simulink library "lib_Convection_ImpingingJet"  (R2015a)
settings: Solver=ode45  StartTime=0.0  StopTime=10.0  RelTol=1e-3
libraries: simulink x35, lib_GenTools_MinMax x1
settings Model: Creator=jlkratz  LastModifiedBy=jlkratz

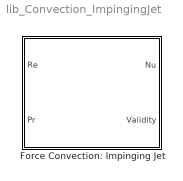
== system lib_Convection_ImpingingJet ==
  Force Convection: Impinging Jet : Subsystem  mask(TSAT: Impinging Jet){RoundOrSlot_M=Slot Nozzle, SingleOrArray_M=Nozzle Array, AlignOrStag_M=Nozzles are aligned, H_M=0.126/12, D_M=0.0625/12, r_M=3, S_M=0.25/12}
      mask prompts: H_M "H_M - Distance from the nozzle to the impingement surface (H)"; D_M "D_M - Diameter of the nozzle (D) for round nozzles or the width of the slot nozzle (W) for slot nozzles"; r_M "r_M - Distance from the stagnation point over which the average Nu is desired (r or x)"; S_M "S_M - Pitch of the array (distance between centerpoints the nozzles in an array)"
      mask help:
      | This block estimates the average Nusselt number for an impinging jet on a surfaces. The implemented correlations were developed by Martin. It is presumed in these correlations that the gas jet exits its nozzle with a uniform velocity, temperature, and species concentration. Thermal and compositional equilibrium with the ambient air are presumed. Conditions are assumed to be uninfluenced by the amount of turbulence at the nozzles and the surface is presumed to be stationary. Fluid properties should be evaluated at the conditions of the jet. This block considers round nozzles, and slot nozzles. It also considers a single nozzle or an array of nozzles. The characteristic length is the hydraulic diameter of the nozzle which happens to be the diameter (D) for round nozzles and 2 times the width of the slot (W) for slot nozzles. The implemented correlations are subject to the following restrictions:
      |
      | Single Round Nozzle:
      | 2000 <= Re <= 400000
      | 2 <= H/D <= 12
      | 0.004 <= Ar <= 0.04
      |
      | Array of Round Nozzles:
      | 2000 <= Re <= 100000
      | 2 <= H/D <= 12
      | 0.004 <= Ar <= 0.04
      |
      | Single Slot Nozzle:
      | 3000 <= Re <= 90000
      | 2 <= H/W <= 10
      | 0.025 <= Ar <= 0.125
      |
      | Array of Slot Nozzles:
      | 1500 <= Re <= 40000
      | 2 <= H/W <= 80
      | 0.008 <= Ar <= 2.5*Aro (Aro is defined in the help menu)
      |
      | Note that Re is the Reynolds number, Pr is the Prandtl number, H is the distance from the nozzle to the impingment surface, and Ar is a nozzle ratio (the nozzle exit area to the surface area of the cell). For a single nozzle the cell is defined by a radius or distance from the stagnation point which defines the area over which the average Nusselt number is to be calculated for. For nozzle areas, the cell area is equally divided area in which each nozzle resides. For more information see the block help menu.
      mask Help: web(which('Convection_TSAT_ImpingingJet.html'),'-helpbrowser')
      mask TypeOptions RoundOrSlot_M: Round Nozzle | Slot Nozzle
      mask Callback RoundOrSlot_M:
      | sel1 = get_param(gcb,'RoundOrSlot_M');
      | sel2 = get_param(gcb,'SingleOrArray_M');
      | if sel2(1) == 'N'
      |     if sel1(1) == 'R'
      |         MSK_SEC_Enables3_TSAT('on',[3],'en')
      |     elseif sel1(1) == 'S'
      |         MSK_SEC_Enables3_TSAT('on',[3],'dis')
      |     end
      | end
      | clear sel1 sel2
      mask TypeOptions SingleOrArray_M: Single Nozzle | Nozzle Array
      mask Callback SingleOrArray_M:
      | sel1 = get_param(gcb,'SingleOrArray_M');
      | sel2 = get_param(gcb,'RoundOrSlot_M');
      | if sel1(1) == 'S'
      |     MSK_SEC_Enables3_TSAT('on',7,'dis')
      |     MSK_SEC_Enables3_TSAT('on',6,'en')
      |     MSK_SEC_Enables3_TSAT('on',3,'dis')
      | elseif sel1(1) == 'N'
      |     MSK_SEC_Enables3_TSAT('on',7,'en')
      |     MSK_SEC_Enables3_TSAT('on',6,'dis')
      |     if sel2(1) == 'R'
      |         MSK_SEC_Enables3_TSAT('on',3,'en')
      |     elseif sel2(1) == 'S'
      |         MSK_SEC_Enables3_TSAT('on',3,'dis')
      |     end
      | end
      | clear sel1 sel2
      mask TypeOptions AlignOrStag_M: Nozzles are aligned | Nozzles are staggered
      mask DialogControl Container3 Prompt: Parameters

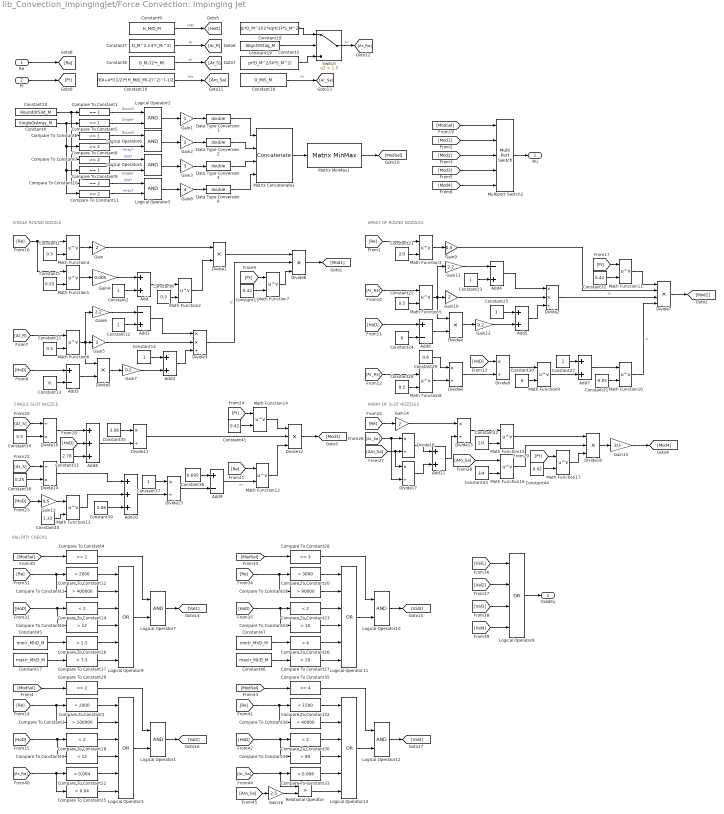
== system lib_Convection_ImpingingJet/Force Convection: Impinging Jet ==
  note: SINGLE ROUND NOZZLE
  note: SINGLE SLOT NOZZLE
  note: ARRAY OF ROUND NOZZLES
  note: ARRAY OF SLOT NOZZLES
  note: VALIDITY CHECKS
  Re : Inport
  Pr : Inport  Port=2
  Add{,2,5,7,11} (5 alike) : Sum
  Add1 : Sum  Inputs=-+
  Add10 : Sum  Inputs=+++
  Add3 : Sum  Inputs=+-
  Add4 : Sum  Inputs=-+
  Add6 : Sum  Inputs=+-
  Add8 : Sum  Inputs=+++
  Add9 : Sum  Inputs=+-
  Compare To Constant{1,4..6,9} (5 alike) : simulink/Logic and Bit Operations/Compare To Constant  relop===  const=1  OutDataTypeStr=boolean
  Compare To Constant{7..8,10..11,29} (5 alike) : simulink/Logic and Bit Operations/Compare To Constant  relop===  const=2  OutDataTypeStr=boolean
  Compare To Constant12 : simulink/Logic and Bit Operations/Compare To Constant  relop=<  const=2000  OutDataTypeStr=boolean
  Compare To Constant13 : simulink/Logic and Bit Operations/Compare To Constant  relop=>  const=400000  OutDataTypeStr=boolean
  Compare To Constant{14,18,23,30} (4 alike) : simulink/Logic and Bit Operations/Compare To Constant  relop=<  const=2  OutDataTypeStr=boolean
  Compare To Constant15 : simulink/Logic and Bit Operations/Compare To Constant  relop=>  const=12  OutDataTypeStr=boolean
  Compare To Constant16 : simulink/Logic and Bit Operations/Compare To Constant  relop=<  const=2.5  OutDataTypeStr=boolean
  Compare To Constant17 : simulink/Logic and Bit Operations/Compare To Constant  relop=>  const=7.5  OutDataTypeStr=boolean
  Compare To Constant19 : simulink/Logic and Bit Operations/Compare To Constant  relop=>  const=12  OutDataTypeStr=boolean
  Compare To Constant2 : simulink/Logic and Bit Operations/Compare To Constant  relop=<  const=2000  OutDataTypeStr=boolean
  Compare To Constant20 : simulink/Logic and Bit Operations/Compare To Constant  relop=<  const=3000  OutDataTypeStr=boolean
  Compare To Constant21 : simulink/Logic and Bit Operations/Compare To Constant  relop=>  const=90000  OutDataTypeStr=boolean
  Compare To Constant22 : simulink/Logic and Bit Operations/Compare To Constant  relop=<  const=0.004  OutDataTypeStr=boolean
  Compare To Constant24 : simulink/Logic and Bit Operations/Compare To Constant  relop=>  const=10  OutDataTypeStr=boolean
  Compare To Constant25 : simulink/Logic and Bit Operations/Compare To Constant  relop=>  const=0.04  OutDataTypeStr=boolean
  Compare To Constant26 : simulink/Logic and Bit Operations/Compare To Constant  relop=<  const=4  OutDataTypeStr=boolean
  Compare To Constant27 : simulink/Logic and Bit Operations/Compare To Constant  relop=>  const=20  OutDataTypeStr=boolean
  Compare To Constant28 : simulink/Logic and Bit Operations/Compare To Constant  relop===  const=3  OutDataTypeStr=boolean
  Compare To Constant3 : simulink/Logic and Bit Operations/Compare To Constant  relop=>  const=100000  OutDataTypeStr=boolean
  Compare To Constant31 : simulink/Logic and Bit Operations/Compare To Constant  relop=>  const=80  OutDataTypeStr=boolean
  Compare To Constant32 : simulink/Logic and Bit Operations/Compare To Constant  relop=<  const=1500  OutDataTypeStr=boolean
  Compare To Constant33 : simulink/Logic and Bit Operations/Compare To Constant  relop=<  const=0.008  OutDataTypeStr=boolean
  Compare To Constant35 : simulink/Logic and Bit Operations/Compare To Constant  relop===  const=4  OutDataTypeStr=boolean
  Compare To Constant36 : simulink/Logic and Bit Operations/Compare To Constant  relop=>  const=40000  OutDataTypeStr=boolean
  Constant{1,6,11,22,28,34} (6 alike) : Constant  Value=0.5
  Constant10 : Constant  Value=(60+4*((1/2)*(H_M/D_M)-2)^2)^(-1/2)
  Constant{2,12,14,23,25,27,37} (7 alike) : Constant
  Constant13 : Constant  Value=6
  Constant{15,32,41,44} (4 alike) : Constant  Value=0.42
  Constant16 : Constant  Value=D_M/S_M
  Constant17 : Constant  Value=max(r_M)/D_M
  Constant18 : Constant  Value=pi*D_M^2/(2*sqrt(3)*S_M^2)
  Constant19 : Constant  Value=AlignOrStag_M
  Constant20 : Constant  Value=RoundOrSlot_M
  Constant21 : Constant  Value=2/3
  Constant24 : Constant  Value=6
  Constant29 : Constant  Value=0.6
  Constant3 : Constant  Value=pi*D_M^2/(4*S_M^2)
  Constant30 : Constant  Value=6
  Constant31 : Constant  Value=-0.05
  Constant33 : Constant  Value=2.78
  Constant35 : Constant  Value=3.06
  Constant36 : Constant  Value=0.695
  Constant38 : Constant  Value=0.25
  Constant39 : Constant  Value=3.06
  Constant4 : Constant  Value=SingleOrArray_M
  Constant40 : Constant  Value=1.33
  Constant42 : Constant  Value=2/3
  Constant43 : Constant  Value=3/4
  Constant45 : Constant  Value=min(r_M)/D_M
  Constant46 : Constant  Value=max(r_M)/D_M
  Constant47 : Constant  Value=min(r_M)/D_M
  Constant5 : Constant  Value=0.55
  Constant7 : Constant  Value=D_M^2./(4*r_M.^2)
  Constant8 : Constant  Value=D_M./(2*r_M)
  Constant9 : Constant  Value=H_M/D_M
  Data Type Conversion{1..3,8} (4 alike) : DataTypeConversion  OutDataTypeStr=double
  Divide1 : Product  Inputs=**
  Divide10 : Product  Inputs=/*
  Divide{8..9,11,13,15..17} (7 alike) : Product  Inputs=*/
  Divide12 : Product  Inputs=***
  Divide14 : Product  Inputs=/*
  Divide18 : Product  Inputs=***
  Divide2 : Product  Inputs=**/
  Divide3 : Product  Inputs=**/
  Divide4 : Product  Inputs=**
  Divide5 : Product  Inputs=**
  Divide6 : Product  Inputs=***
  Divide7 : Product  Inputs=****
  Gain{,2,5,10,14} (5 alike) : Gain  Gain=2
  Gain1 : Gain
  Gain11 : Gain  Gain=2.2
  Gain12 : Gain  Gain=0.2
  Gain13 : Gain  Gain=0.5
  Gain15 : Gain  Gain=2/3
  Gain16 : Gain  Gain=2.5
  Gain3 : Gain  Gain=3
  Gain4 : Gain  Gain=0.005
  Gain6 : Gain  Gain=2.2
  Gain7 : Gain  Gain=0.2
  Gain8 : Gain  Gain=4
  Gain9 : Gain  Gain=0.5
  Logical Operator{1..2,4..7,10,12} (8 alike) : Logic  AllPortsSameDT=off  OutDataTypeStr=boolean
  Logical Operator{3,9,11,13} (4 alike) : Logic  Operator=OR  Inputs=6  AllPortsSameDT=off  OutDataTypeStr=boolean
  Logical Operator8 : Logic  Operator=OR  Inputs=4  AllPortsSameDT=off  OutDataTypeStr=boolean
  Math Function{1..17} (17 alike) : Math  Operator=pow  SaturateOnIntegerOverflow=on
  Matrix Concatenate1 : Concatenate  NumInputs=4  Mode=Multidimensional array  ConcatenateDimension=2
  Matrix MinMax1 : lib_GenTools_MinMax/Matrix MinMax  rows_M=on  cols_M=off  all_M=off  minmax_M=off  BN_M=gcb
  Multiport Switch2 : MultiPortSwitch  Inputs=4
  Relational Operator : RelationalOperator  Operator=>  OutDataTypeStr=boolean
  Switch : Switch  Criteria=u2 > Threshold  Threshold=1.5
  Nu : Outport
  Validity : Outport  Port=2
  wires:
  Gain16/1 -> Relational Operator/2
  Constant1/1 -> Math Function4/2
  Re/1 -> [Re]
  Pr/1 -> [Pr]
  [ModSel] -> Multiport Switch2/1
  Multiport Switch2/1 -> Nu/1
  Matrix MinMax1/1 -> [ModSel]
  Matrix Concatenate1/1 -> Matrix MinMax1/1
  [Re] -> Math Function1/1, Math Function4/1
  Gain1/1 -> Data Type Conversion1/1
  Logical Operator2/1 -> Gain1/1
  Gain2/1 -> Data Type Conversion2/1
  Logical Operator6/1 -> Gain2/1
  Gain3/1 -> Data Type Conversion3/1
  Logical Operator4/1 -> Gain3/1
  Gain8/1 -> Data Type Conversion8/1
  Logical Operator5/1 -> Gain8/1
  Data Type Conversion1/1 -> Matrix Concatenate1/1
  Data Type Conversion2/1 -> Matrix Concatenate1/2
  Data Type Conversion3/1 -> Matrix Concatenate1/3
  Data Type Conversion8/1 -> Matrix Concatenate1/4
  Constant20/1 -> Compare To Constant10/1, Compare To Constant7/1, Compare To Constant6/1, Compare To Constant1/1
  Constant4/1 -> Compare To Constant11/1, Compare To Constant9/1, Compare To Constant8/1, Compare To Constant5/1
  Compare To Constant1/1 -> Logical Operator2/1  "Round?"
  Compare To Constant5/1 -> Logical Operator2/2  "Single?"
  Compare To Constant6/1 -> Logical Operator6/1  "Round?"
  Compare To Constant8/1 -> Logical Operator6/2  "Array?"
  Compare To Constant7/1 -> Logical Operator4/1  "Slot?"
  Compare To Constant9/1 -> Logical Operator4/2  "Single?"
  Compare To Constant10/1 -> Logical Operator5/1  "Slot?"
  Compare To Constant11/1 -> Logical Operator5/2  "Array?"
  [Mod1] -> Multiport Switch2/2
  [Mod2] -> Multiport Switch2/3
  [Mod3] -> Multiport Switch2/4
  [Mod4] -> Multiport Switch2/5
  Math Function4/1 -> Gain/1
  Constant2/1 -> Add/2
  Constant5/1 -> Math Function1/2
  Math Function1/1 -> Gain4/1
  Gain4/1 -> Add/1
  Add/1 -> Math Function2/1
  Constant6/1 -> Math Function2/2
  Math Function2/1 -> Divide1/2
  Gain/1 -> Divide1/1
  Constant7/1 -> [Ar_R]  "Ar"
  Constant8/1 -> [Ar_S]  "Ar"
  Constant9/1 -> [HoD]  "H/D"
  Constant10/1 -> [Aro_Sa]  "Aro"
  [Ar_R] -> Math Function6/1
  Constant11/1 -> Math Function6/2
  Math Function6/1 -> Divide5/1, Gain6/1, Gain5/1
  Constant12/1 -> Add1/2
  Gain6/1 -> Add1/1
  Gain5/1 -> Divide3/2
  Add1/1 -> Divide3/1
  [HoD] -> Add3/1
  Constant13/1 -> Add3/2
  Add3/1 -> Divide5/2
  Divide5/1 -> Gain7/1
  Gain7/1 -> Add2/2
  Constant14/1 -> Add2/1
  Add2/1 -> Divide3/3
  Divide1/1 -> Divide6/1
  Divide3/1 -> Divide6/2  "G"
  [Pr] -> Math Function7/1
  Math Function7/1 -> Divide6/3
  Constant15/1 -> Math Function7/2
  Divide6/1 -> [Mod1]
  Constant16/1 -> [Ar_Sa]  "Ar"
  Constant3/1 -> Switch/3
  Constant18/1 -> Switch/1
  Switch/1 -> [Ar_Ra]  "Ar"
  Constant19/1 -> Switch/2
  Constant21/1 -> Math Function3/2
  [Re] -> Math Function3/1
  Math Function3/1 -> Gain9/1
  Gain9/1 -> Divide7/2
  [Ar_Ra] -> Math Function5/1
  Constant22/1 -> Math Function5/2
  Math Function5/1 -> Gain10/1, Gain11/1, Divide4/1
  Constant23/1 -> Add4/2
  Gain11/1 -> Add4/1
  Gain10/1 -> Divide2/2
  Add4/1 -> Divide2/1
  [HoD] -> Add6/1
  Add6/1 -> Divide4/2
  Divide4/1 -> Gain12/1
  Gain12/1 -> Add5/2
  Constant25/1 -> Add5/1
  Add5/1 -> Divide2/3
  Divide2/1 -> Divide7/3  "G"
  Constant24/1 -> Add6/2
  Math Function9/1 -> Add7/2
  Constant27/1 -> Add7/1
  [Ar_Ra] -> Math Function8/1
  Constant28/1 -> Math Function8/2
  Math Function8/1 -> Divide8/2
  Constant29/1 -> Divide8/1
  Divide8/1 -> Divide9/2
  [HoD] -> Divide9/1
  Divide9/1 -> Math Function9/1
  Constant30/1 -> Math Function9/2
  Add7/1 -> Math Function10/1
  Constant31/1 -> Math Function10/2
  Math Function10/1 -> Divide7/4  "K"
  Divide7/1 -> [Mod2]
  [Pr] -> Math Function11/1
  Math Function11/1 -> Divide7/1
  Constant32/1 -> Math Function11/2
  Constant34/1 -> Divide10/2
  [Ar_S] -> Divide10/1
  Divide10/1 -> Add8/1
  [HoD] -> Add8/2
  Constant33/1 -> Add8/3
  Add8/1 -> Divide11/2
  Constant35/1 -> Divide11/1
  [Re] -> Math Function12/1
  Add9/1 -> Math Function12/2  "m"
  Divide11/1 -> Divide12/2
  Math Function12/1 -> Divide12/3
  Divide12/1 -> [Mod3]
  Constant37/1 -> Divide13/1
  Constant36/1 -> Add9/1
  Divide13/1 -> Add9/2
  Add10/1 -> Divide13/2
  Constant38/1 -> Divide14/2
  [Ar_S] -> Divide14/1
  Constant39/1 -> Add10/3
  Divide14/1 -> Add10/1
  [HoD] -> Gain13/1
  Gain13/1 -> Math Function13/1
  Constant40/1 -> Math Function13/2
  Math Function13/1 -> Add10/2
  [Pr] -> Math Function14/1
  Math Function14/1 -> Divide12/1
  Constant41/1 -> Math Function14/2
  [Re] -> Gain14/1
  [Ar_Sa] -> Divide17/2, Divide16/1
  [Aro_Sa] -> Divide17/1, Divide16/2
  Divide16/1 -> Add11/1
  Divide17/1 -> Add11/2
  Gain14/1 -> Divide15/1
  Add11/1 -> Divide15/2
  Divide15/1 -> Math Function15/1
  Constant42/1 -> Math Function15/2
  [Aro_Sa] -> Math Function16/1
  Constant43/1 -> Math Function16/2
  Math Function15/1 -> Divide18/1
  Math Function16/1 -> Divide18/2
  [Pr] -> Math Function17/1
  Constant44/1 -> Math Function17/2
  Math Function17/1 -> Divide18/3
  Divide18/1 -> Gain15/1
  Gain15/1 -> [Mod4]
  [Re] -> Compare To Constant13/1, Compare To Constant12/1
  [HoD] -> Compare To Constant15/1, Compare To Constant14/1
  Constant45/1 -> Compare To Constant16/1
  Constant17/1 -> Compare To Constant17/1
  Compare To Constant16/1 -> Logical Operator9/5
  Compare To Constant17/1 -> Logical Operator9/6
  Compare To Constant15/1 -> Logical Operator9/4
  Compare To Constant14/1 -> Logical Operator9/3
  Compare To Constant13/1 -> Logical Operator9/2
  Compare To Constant12/1 -> Logical Operator9/1
  [ModSel] -> Compare To Constant4/1
  Logical Operator9/1 -> Logical Operator7/2
  Compare To Constant4/1 -> Logical Operator7/1
  [Re] -> Compare To Constant20/1, Compare To Constant21/1
  [HoD] -> Compare To Constant23/1, Compare To Constant24/1
  Constant47/1 -> Compare To Constant26/1
  Constant46/1 -> Compare To Constant27/1
  Compare To Constant26/1 -> Logical Operator11/5
  Compare To Constant27/1 -> Logical Operator11/6
  Compare To Constant24/1 -> Logical Operator11/4
  Compare To Constant23/1 -> Logical Operator11/3
  Compare To Constant21/1 -> Logical Operator11/2
  Compare To Constant20/1 -> Logical Operator11/1
  [ModSel] -> Compare To Constant28/1
  Logical Operator11/1 -> Logical Operator10/2
  Compare To Constant28/1 -> Logical Operator10/1
  Logical Operator8/1 -> Validity/1
  Logical Operator7/1 -> [Val1]
  Logical Operator10/1 -> [Val3]
  [Val1] -> Logical Operator8/1
  [Val2] -> Logical Operator8/2
  [Val3] -> Logical Operator8/3
  [Val4] -> Logical Operator8/4
  [Re] -> Compare To Constant2/1, Compare To Constant3/1
  [HoD] -> Compare To Constant18/1, Compare To Constant19/1
  [Ar_Ra] -> Compare To Constant25/1, Compare To Constant22/1
  Compare To Constant22/1 -> Logical Operator3/5
  Compare To Constant25/1 -> Logical Operator3/6
  Compare To Constant19/1 -> Logical Operator3/4
  Compare To Constant18/1 -> Logical Operator3/3
  Compare To Constant3/1 -> Logical Operator3/2
  Compare To Constant2/1 -> Logical Operator3/1
  [ModSel] -> Compare To Constant29/1
  Logical Operator3/1 -> Logical Operator1/2
  Compare To Constant29/1 -> Logical Operator1/1
  Logical Operator1/1 -> [Val2]
  [Re] -> Compare To Constant36/1, Compare To Constant32/1
  [HoD] -> Compare To Constant31/1, Compare To Constant30/1
  [Ar_Sa] -> Relational Operator/1, Compare To Constant33/1
  Compare To Constant33/1 -> Logical Operator13/5
  Relational Operator/1 -> Logical Operator13/6
  Compare To Constant31/1 -> Logical Operator13/4
  Compare To Constant30/1 -> Logical Operator13/3
  Compare To Constant36/1 -> Logical Operator13/2
  Compare To Constant32/1 -> Logical Operator13/1
  [ModSel] -> Compare To Constant35/1
  Logical Operator13/1 -> Logical Operator12/2
  Compare To Constant35/1 -> Logical Operator12/1
  Logical Operator12/1 -> [Val4]
  [Aro_Sa] -> Gain16/1
